simulink model "rectangular"  (R2024b)
settings: Solver=ode45  StartTime=0.0  StopTime=10000  FixedStep=0.05  MaxStep=30  RelTol=1e-3
undefined symbols (not defined in the file or in its folder): utrim
settings Model: Creator=rzxha  LastModifiedBy=rzxha

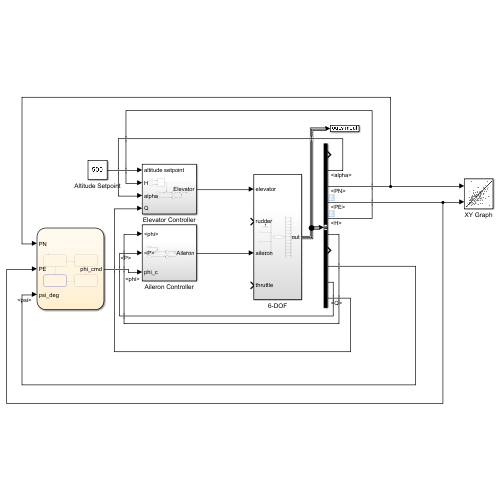
[thumbnail: Simulink's stored preview of the top-level diagram]
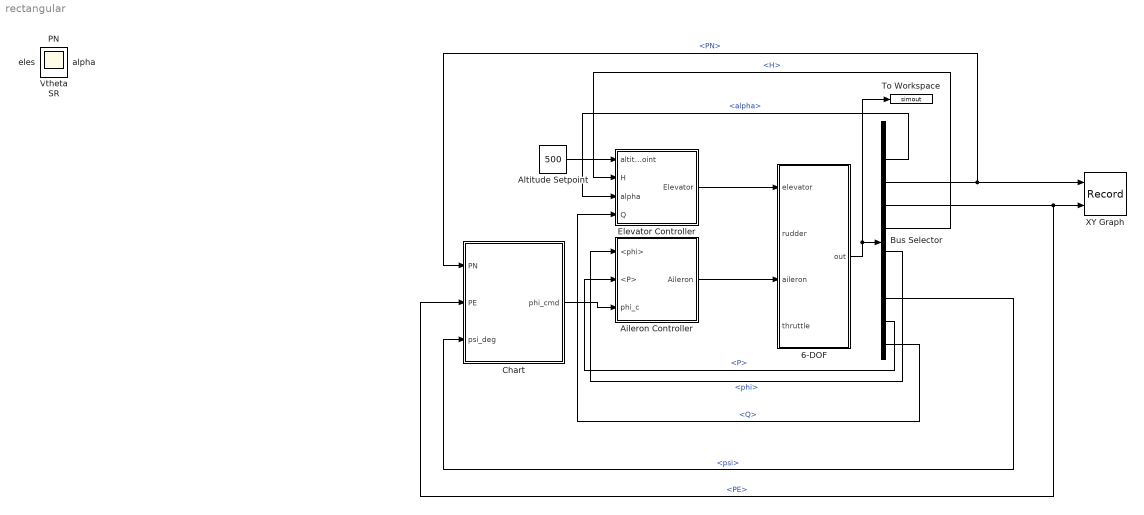
== system rectangular ==
  6-DOF : Subsystem
  Aileron Controller : Subsystem
  Altitude Setpoint : Constant  Value=500
  Bus Selector : BusSelector  OutputSignals=Vt,alpha,PN,PE,H,phi,theta,psi,P,Q
  Chart : Stateflow chart  TreatAsAtomicUnit=on
      settings: PortSchema="{\"entries\":[{\"content\":{\"sides\":[{\"content\":{\"connectorIds\":[\"In3\",\"In2\",\"In1\"]},\"type\":\"ConnectorPlacement.EquallySpacedRectSide\",\"uuid\":\"b63685ba-98bf-4ede-bd7f-b85c64b9efcb\"},{\"content\":{\"connectorIds\":[\"Out1\"],\"side\":\"RIGHT\"},\"type\":\"ConnectorPlacement.EquallySpacedRectSide\",\"uuid\":\"35761f39-ee5e-41e2-91cf-295f71e45681\"},{\"content\":{\"connectorIds\":[],\"side\":\"TOP\"},\"type\":\"ConnectorPlacement.EquallySpacedRectSide\",\"uuid\":\"fc2bdb40-36e9-4955-80e1-5f82893c8815\"}]},\"type\":\"ConnectorPlacement.EquallySpacedConnector\",\"uuid\":\"d080a6f2-4957-4a6a-b923-4309b873cf7c\"}],\"packageUris\":[\"http://schema.mathworks.com/mf0/Connector/R2020b\"],\"version\":\"1.0\"}"
  Elevator Controller : Subsystem
  To Workspace : ToWorkspace  VariableName=simout  SampleTime=-1
  XY Graph : Record  FileSettingsInternal="{\"entries\":[{\"content\":{\"excelSettings\":{\"content\":{},\"type\":\"Streamout.ExcelSettings\"}},\"type\":\"Streamout.FileSettingStorage\",\"uuid\":\"\"}],\"packageUris\":[\"http:\\/\\/schema.mathworks.com\\/mf0\\/streamout_blocks\\/R2020a\"],\"version\":\"1.0\"}"  Layout=[1 1]  SignalsInternal="{\"entries\":[{\"content\":{\"signals\":[{\"content\":{\"blockPath\":[],\"dimensions\":[1],\"domain\":\"\",\"lineColor\":\"#a2142f\",\"plots\":[ 1 ],\"port\":1,\"sid\":[\"\"],\"signalID\":1,\"signalName\":\"<PN>\"},\"type\":\"RecordBlkView.Signal\",\"uuid\":\"\"},{\"content\":{\"blockPath\":[],\"dimensions\":[1],\"domain\":\"\",\"lineColor\":\"#139fff\",\"plots\":[ 1 ],\"port\":2,\"sid\":[\"\"],\"signalID\":2,\"signalName\":\"<PE>\"},\"type\":\"RecordBlkView.Signal\",\"uuid\":\"\"},{\"content\":{\"blockPath\":[],\"dimensions\":[13],\"domain\":\"\",\"hasChildren\":true,\"lineColor\":\"#77ac30\",\"lineWidth\":2,\"port\":1,\"sid\":[\"\"],\"signalID\":3,\"signalName\":\"6-DOF\"},\"type\":\"RecordBlkView.Signal\",\"uuid\":\"\"},{\"content\":{\"blockPath\":[],\"channel\":[1],\"dimensions\":[13],\"domain\":\"\",\"lineColor\":\"#139fff\",\"lineWidth\":2,\"parentID\":3,\"port\":1,\"sid\":[\"\"],\"signalID\":4,\"signalName\":\"6-DOF\"},\"type\":\"RecordBlkView.Signal\",\"uuid\":\"\"}]},\"type\":\"RecordBlkView.InputSignals\",\"uuid\":\"\"}],\"packageUris\":[\"http:\\/\\/schema.mathworks.com\\/mf0\\/streamout_blocks\\/R2020a\"],\"version\":\"1.0\"}"  VisualizationBindings="{\"xyplotplugin\":{\"info\":[{\"series\":[{\"bindingParametersList\":[{\"parameter\":\"X-Axis\",\"signalID\":1,\"signalName\":\"<PN>\"},{\"parameter\":\"Y-Axis\",\"signalID\":2,\"signalName\":\"<PE>\"}],\"seriesID\":0}],\"subplotID\":1}]}}"  CompatibilityTag=XY
  H : Scope
  PN : Scope
  SR : Scope
  Vt : Scope
  alpha : Scope
  eles : Scope
  theta : Scope
  wires:
  Bus Selector/10 -> Elevator Controller/4(Q)  "<Q>"
  Bus Selector/5 -> Elevator Controller/2(H)  "<H>"
  Bus Selector/2 -> Elevator Controller/3(alpha)  "<alpha>"
  Bus Selector/3 -> XY Graph/1, Chart/3(PN)  "<PN>"
  Bus Selector/4 -> XY Graph/2, Chart/2(PE)  "<PE>"
  Aileron Controller/1(Aileron) -> 6-DOF/3(aileron)
  Elevator Controller/1(Elevator) -> 6-DOF/1(elevator)
  Bus Selector/6 -> Aileron Controller/1(<phi>)  "<phi>"
  Bus Selector/8 -> Chart/1(psi_deg)  "<psi>"
  Chart/1(phi_cmd) -> Aileron Controller/3(phi_c)
  Altitude Setpoint/1 -> Elevator Controller/1(altitude setpoint)
  Bus Selector/9 -> Aileron Controller/2(<P>)  "<P>"
  6-DOF/1(out) -> To Workspace/1, Bus Selector/1

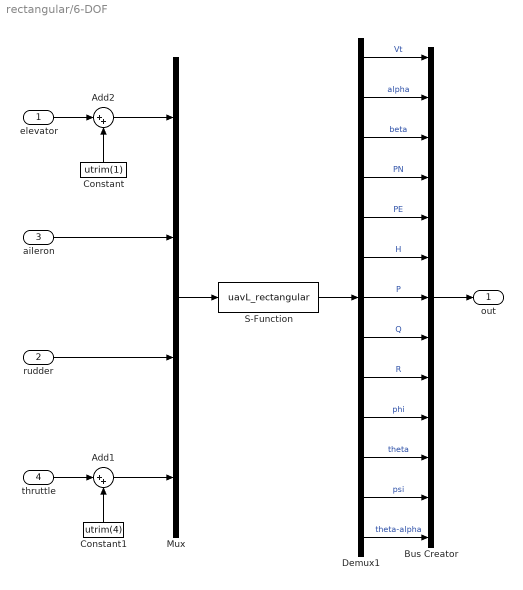
== system rectangular/6-DOF ==
  elevator : Inport
  rudder : Inport  Port=2
  aileron : Inport  Port=3
  thruttle : Inport  Port=4
  Add1 : Sum  Inputs=|++
  Add2 : Sum  Inputs=|++
  Bus Creator : BusCreator  Inputs=13
  Constant : Constant  Value=utrim(1)
  Constant1 : Constant  Value=utrim(4)
  Demux1 : Demux  Outputs=13
  Mux : Mux
  S-Function : S-Function  FunctionName=uavL_rectangular  SFunctionDeploymentMode=off  EnableBusSupport=off
  out : Outport
  wires:
  Demux1/8 -> Bus Creator/8  "Q"
  elevator/1 -> Add2/1
  aileron/1 -> Mux/2
  Constant1/1 -> Add1/2
  Demux1/6 -> Bus Creator/6  "H"
  Constant/1 -> Add2/2
  thruttle/1 -> Add1/1
  Add1/1 -> Mux/4
  rudder/1 -> Mux/3
  Add2/1 -> Mux/1
  Mux/1 -> S-Function/1
  S-Function/1 -> Demux1/1
  Demux1/11 -> Bus Creator/11  "theta"
  Demux1/1 -> Bus Creator/1  "Vt"
  Demux1/13 -> Bus Creator/13  "theta-alpha"
  Demux1/2 -> Bus Creator/2  "alpha"
  Demux1/3 -> Bus Creator/3  "beta"
  Demux1/4 -> Bus Creator/4  "PN"
  Demux1/5 -> Bus Creator/5  "PE"
  Demux1/7 -> Bus Creator/7  "P"
  Demux1/9 -> Bus Creator/9  "R"
  Demux1/10 -> Bus Creator/10  "phi"
  Demux1/12 -> Bus Creator/12  "psi"
  Bus Creator/1 -> out/1

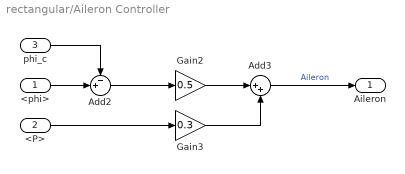
== system rectangular/Aileron Controller ==
  <phi> : Inport
  <P> : Inport  Port=2
  phi_c : Inport  Port=3
  Add2 : Sum  Inputs=-+|
  Add3 : Sum  Inputs=|++
  Gain2 : Gain  Gain=0.5
  Gain3 : Gain  Gain=0.3
  Aileron : Outport
  wires:
  Gain2/1 -> Add3/1
  Gain3/1 -> Add3/2
  Add3/1 -> Aileron/1  "Aileron"
  <phi>/1 -> Add2/2
  Add2/1 -> Gain2/1
  <P>/1 -> Gain3/1
  phi_c/1 -> Add2/1

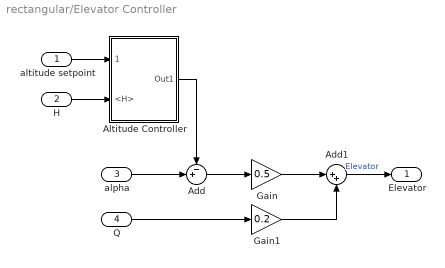
== system rectangular/Elevator Controller ==
  altitude setpoint : Inport
  H : Inport  Port=2
  alpha : Inport  Port=3
  Q : Inport  Port=4
  Add : Sum  Inputs=-+|
  Add1 : Sum  Inputs=|++
  Altitude Controller : Subsystem
  Gain : Gain  Gain=0.5
  Gain1 : Gain  Gain=0.2
  Elevator : Outport
  wires:
  Q/1 -> Gain1/1
  Gain/1 -> Add1/1
  alpha/1 -> Add/2
  Add/1 -> Gain/1
  H/1 -> Altitude Controller/2(<H>)
  Altitude Controller/1(Out1) -> Add/1
  altitude setpoint/1 -> Altitude Controller/1(Altitude Setpoint)
  Gain1/1 -> Add1/2
  Add1/1 -> Elevator/1  "Elevator"

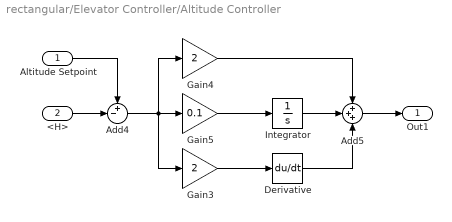
== system rectangular/Elevator Controller/Altitude Controller ==
  Altitude Setpoint : Inport
  <H> : Inport  Port=2
  Add4 : Sum  Inputs=+-|
  Add5 : Sum  Inputs=+++
  Derivative : Derivative
  Gain3 : Gain  Gain=2
  Gain4 : Gain  Gain=2
  Gain5 : Gain  Gain=0.1
  Integrator : Integrator
  Out1 : Outport
  wires:
  Derivative/1 -> Add5/3
  Add4/1 -> Gain4/1, Gain5/1, Gain3/1
  Gain5/1 -> Integrator/1
  Gain3/1 -> Derivative/1
  Altitude Setpoint/1 -> Add4/1
  Add5/1 -> Out1/1
  <H>/1 -> Add4/2
  Integrator/1 -> Add5/2
  Gain4/1 -> Add5/1

== stateflow chart rectangular/Chart ==
  state step1
    entry:psi_cmd=0;
    during:dpsi=psi_cmd-psi_deg;
    while(dpsi>180) dpsi=dpsi-360;end
    while(dpsi<-180) dpsi=dpsi+360;end
    phi_cmd=1.0*dpsi;
    if(phi_cmd>45) phi_cmd=45;end
    if(phi_cmd<-45) phi_cmd=-45;end
  state step2
    entry:psi_cmd=90;
    during:dpsi=psi_cmd-psi_deg;
    while(dpsi>180) dpsi=dpsi-360;end
    while(dpsi<-180) dpsi=dpsi+360;end
    phi_cmd=1.0*dpsi;
    if(phi_cmd>45) phi_cmd=45;end
    if(phi_cmd<-45) phi_cmd=-45;end
  state step4
    entry:psi_cmd=270;
    during:dpsi=psi_cmd-psi_deg;
    while(dpsi>180) dpsi=dpsi-360;end
    while(dpsi<-180) dpsi=dpsi+360;end
    phi_cmd=1.0*dpsi;
    if(phi_cmd>45) phi_cmd=45;end
    if(phi_cmd<-45) phi_cmd=-45;end
  state step3
    entry:psi_cmd=180;
    during:dpsi=psi_cmd-psi_deg;
    while(dpsi>180) dpsi=dpsi-360;end
    while(dpsi<-180) dpsi=dpsi+360;end
    phi_cmd=1.0*dpsi;
    if(phi_cmd>45) phi_cmd=45;end
    if(phi_cmd<-45) phi_cmd=-45;end
  (default) -> step1
  step1 -> step2 : [PN>1000]
  step4 -> step1 : [PE<0]
  step2 -> step3 : [PE>1000]
  step3 -> step4 : [PN<0]
  data: phi_cmd output; psi_cmd local; dpsi local; psi_deg input; PE input; PN input
